simulink model "successPIDClosedLoop20picont"  (R2023b)
settings: Solver=FixedStepAuto  StartTime=0.0  StopTime=inf  RelTol=1e-3  EnableMultiTasking=on
libraries: arduinolib x5, simulink x1, arduinosensorlib x1, slpidlib x1
(part 2 of 3)

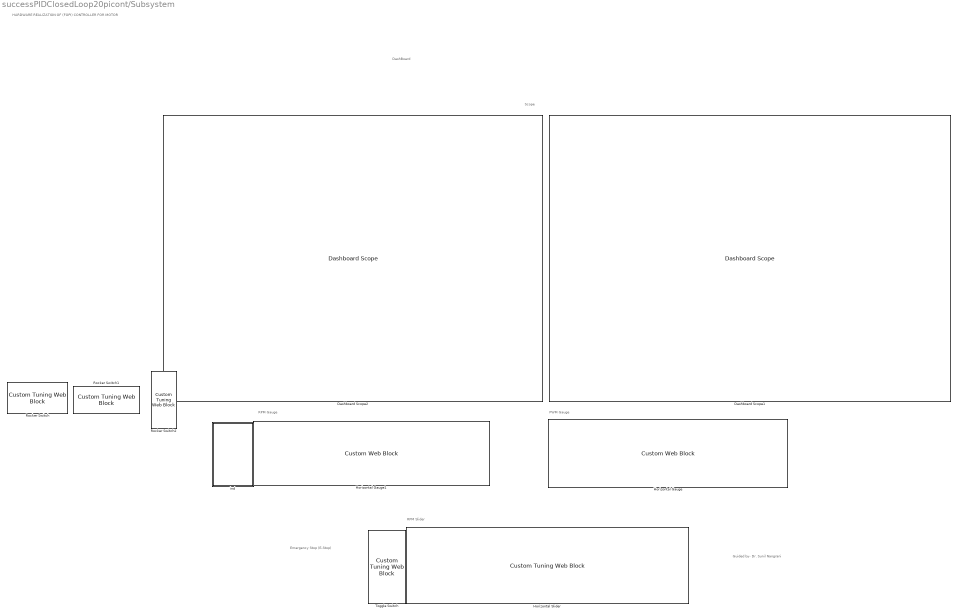
== system successPIDClosedLoop20picont/Subsystem ==
  note: PWM Gauge
  note: RPM Slider
  note: RPM Gauge
  note: Emergency Stop (E-Stop)
  note: DashBoard
  note: Scope
  note: Guided by-
      | Dr. Sunil Nangrani
  note: HARDWARE REALIZATION OF (FOPI) CONTROLLER FOR MOTOR
  Dashboard Scope1 : DashboardScope  UpdateMode=Scroll
  Dashboard Scope2 : DashboardScope  UpdateMode=Scroll
  Horizontal Gauge : CustomWebBlock  LabelPosition=Hide  ShowInitialText=on  Configuration="{\"components\":[{\"name\":\"LinearScaleComponent\",\"settings\":{\"bounds\":{\"max\":1000,\"min\":0,\"tickInterval\":\"auto\"},\"internalTickHeightScaleFactor\":0.5,\"labelColor\":[255,255,200],\"labelFont\":{\"font\":\"Arial\",\"fontSize\":12},\"labelOffset\":0.05,\"labelTransparency\":1,\"needleImage\":{\"size\":[21,75],\"src\":\"data:image\\/svg+xml;base64,PHN2ZyB4bWxucz0iaHR0cDovL3d3dy53My5vcmcvMjAwMC9zdmciIHhtbG5zOnhsaW5rPSJodHRwOi8vd3d3LnczLm9yZy8xOTk5L3hsaW5rIiB2aWV3Qm94PSIwIDAgMjEgNzUiPjxkZWZzPjxzdHlsZT4uY2xzLTF7ZmlsbDpub25lO30uY2xzLTJ7aXNvbGF0aW9uOmlzb2xhdGU7fS5jbHMtM3tjbGlwLXBhdGg6dXJsKCNjbGlwLXBhdGgpO30uY2xzLTR7b3BhY2l0eTowLjM7bWl4LWJsZW5kLW1vZGU6bXVsdGlwbHk7fS5jbHMtNXtmaWxsOiNlYjI2Mjk7fTwvc3R5bGU+PGNsaXBQYXRoIGlkPSJjbGlwLXBhdGgiIHRyYW5zZm9y ...(+1928 chars)\",\"srcOrientation\":\"Right\"},\"needleOffset\":[0.046142754145638065,0.04208955223880597],\"needleSize\":{\"height\":0.7998846597462514,\"width\":0.12797982885085574},\"position\":[0.06969246031746032,0.01995798319327731,0.9641544117647058,0.7998511904761905],\"referencePoint\":\"auto\",\"scaleColors\":[],\"scaleColorsSize\":0.2,\"scaleDirection\":\"LR\",\"showLabels\":1,\"showMinorTicks\":0,\"showSpanLine\":1,\"showTicks\":1,\"tickColor\":[252,252,197],\"tickTransparency\":1,\"valueBarColor\":[23,89,176],\"valueBarOffset\":0,\"valueBarSize\":0.23,\"valueBarTransparency\":1}},{\"name\":\"BackgroundImageComponent\",\"settings\":{\"image\":{\"size\":[380,101],\"src\":\"data:image\\/svg+xml;base64,PHN2ZyBpZD0iZnJhbWUiIHhtbG5zPSJodHRwOi8vd3d3LnczLm9yZy8yMDAwL3N2ZyIgeG1sbnM6eGxpbms9Imh0dHA6Ly93d3cudzMub3JnLzE5OTkveGxpbmsiIHZpZXdCb3g9IjAgMCAzODAgMTAxIj48ZGVmcz48c3R5bGU+LmNscy0xe2ZpbGw6IzAwMmI0Mjt9LmNscy0ye2ZpbGw6IzQyNzA4Mjt9LmNscy0ze2ZpbGw6dXJsKCNyYWRpYWwtZ3JhZGllbnQpO308L3N0eWxlPjxyYWRpYWxHcmFkaWVudCBpZD0icmFkaWFsLWdyYWRpZW50IiBjeD0iMTkwIiBjeT0iNTAuNSIgcj0iMjY5LjIxIiBncmFkaWVudFVuaXRzPSJ1c2VyU3BhY2VPblVzZSI+PHN0b3Agb2Zmc2V0PSIwLjAxIiBzdG9wLWNvbG9yPSIjM2U0ZjU4Ii8+PHN0b3Agb2Zmc2V0PSIwLjA2IiBzdG9wLWNvbG9yPSIjNDQ1NzYxIi8+PHN0b3Agb2Zmc2V0PSIwLjE1IiBzdG9wLWNvbG9yPSIjNTU2YTc2Ii8+PHN0b3Agb2Zmc2V0PSIwLjI1IiBzdG9wLWNvbG9yPSIjNmQ4ODk1Ii8+PHN0b3Agb2Zmc2V0PSIwLjM4IiBzdG9wLWNvbG9yPSIjOGZiMmMzIi8+PHN0b3Agb2Zmc2V0PSIwLjUyIiBzdG9wLWNvbG9yPSIjYjZlNGZhIi8+PHN0b3Agb2Zmc2V0PSIxIiBzdG9wLWNvbG9yPSIjMTU0NjU3Ii8+PC9yYWRpYWxHcmFkaWVudD48L2RlZnM+PGcgaWQ9IkxheWVyXzIiIGRhdGEtbmFtZT0iTGF5ZXIgMiI+PGcgaWQ9IkxheWVyXzEtMiIgZGF0YS1uYW1lPSJMYXllciAxLTIiPjxyZWN0IGlkPSJyZWN0MTAzNiIgY2xhc3M9ImNscy0xIiB4PSIxMSIgeT0iMTEiIHdpZHRoPSIzNTgiIGhlaWdodD0iNzkiLz48cGF0aCBpZD0icGF0aDEwMzgiIGNsYXNzPSJjbHMtMiIgZD0iTTgsOFY5M0gzNzJWOFpNMzY5LDkwSDExVjExSDM2OVoiLz48cGF0aCBpZD0icGF0aDEwNDAiIGNsYXNzPSJjbHMtMyIgZD0iTTAsMFYxMDFIMzgwVjBaTTM3Miw5M0g4VjhIMzcyWiIvPjwvZz48L2c+PC9zdmc+\",\"srcOrientation\":\"horizontal\"},\"position\":[0,0,1,1],\"scaleMode\":\"0\"}},{\"name\":\"ForegroundImageComponent\",\"settings\":{\"image\":{\"size\":[0,0],\"src\":\"default\",\"srcOrientation\":[]},\"isForeground\":1,\"position\":[0,0,1,1],\"scaleMode\":\"0\"}}],\"settings\":{\"BindingType\":\"signal\",\"backgroundColor\":[0,0,0,\"1\"],\"backgroundOffset\":0,\"backgroundOpacity\":1,\"fixedAspectRatio\":\"on\",\"orientation\":\"horizontal\",\"showBackgroundColor\":false,\"value\":0,\"version\":\"R2023a\"},\"type\":\"LinearGauge\"}"
  Horizontal Gauge1 : CustomWebBlock  LabelPosition=Hide  ShowInitialText=on  Configuration="{\"components\":[{\"name\":\"LinearScaleComponent\",\"settings\":{\"bounds\":{\"max\":1000,\"min\":0,\"tickInterval\":\"auto\"},\"internalTickHeightScaleFactor\":0.5,\"labelColor\":[255,255,200],\"labelFont\":{\"font\":\"Arial\",\"fontSize\":12},\"labelOffset\":0.05,\"labelTransparency\":1,\"needleImage\":{\"size\":[21,75],\"src\":\"data:image\\/svg+xml;base64,PHN2ZyB4bWxucz0iaHR0cDovL3d3dy53My5vcmcvMjAwMC9zdmciIHhtbG5zOnhsaW5rPSJodHRwOi8vd3d3LnczLm9yZy8xOTk5L3hsaW5rIiB2aWV3Qm94PSIwIDAgMjEgNzUiPjxkZWZzPjxzdHlsZT4uY2xzLTF7ZmlsbDpub25lO30uY2xzLTJ7aXNvbGF0aW9uOmlzb2xhdGU7fS5jbHMtM3tjbGlwLXBhdGg6dXJsKCNjbGlwLXBhdGgpO30uY2xzLTR7b3BhY2l0eTowLjM7bWl4LWJsZW5kLW1vZGU6bXVsdGlwbHk7fS5jbHMtNXtmaWxsOiNlYjI2Mjk7fTwvc3R5bGU+PGNsaXBQYXRoIGlkPSJjbGlwLXBhdGgiIHRyYW5zZm9y ...(+1928 chars)\",\"srcOrientation\":\"Right\"},\"needleOffset\":[0.046142754145638065,0.04208955223880597],\"needleSize\":{\"height\":0.7998846597462514,\"width\":0.12797982885085574},\"position\":[0.06969246031746032,0.01995798319327731,0.9641544117647058,0.7998511904761905],\"referencePoint\":\"auto\",\"scaleColors\":[],\"scaleColorsSize\":0.2,\"scaleDirection\":\"LR\",\"showLabels\":1,\"showMinorTicks\":0,\"showSpanLine\":1,\"showTicks\":1,\"tickColor\":[252,252,197],\"tickTransparency\":1,\"valueBarColor\":[23,89,176],\"valueBarOffset\":0,\"valueBarSize\":0.23,\"valueBarTransparency\":1}},{\"name\":\"BackgroundImageComponent\",\"settings\":{\"image\":{\"size\":[380,101],\"src\":\"data:image\\/svg+xml;base64,PHN2ZyBpZD0iZnJhbWUiIHhtbG5zPSJodHRwOi8vd3d3LnczLm9yZy8yMDAwL3N2ZyIgeG1sbnM6eGxpbms9Imh0dHA6Ly93d3cudzMub3JnLzE5OTkveGxpbmsiIHZpZXdCb3g9IjAgMCAzODAgMTAxIj48ZGVmcz48c3R5bGU+LmNscy0xe2ZpbGw6IzAwMmI0Mjt9LmNscy0ye2ZpbGw6IzQyNzA4Mjt9LmNscy0ze2ZpbGw6dXJsKCNyYWRpYWwtZ3JhZGllbnQpO308L3N0eWxlPjxyYWRpYWxHcmFkaWVudCBpZD0icmFkaWFsLWdyYWRpZW50IiBjeD0iMTkwIiBjeT0iNTAuNSIgcj0iMjY5LjIxIiBncmFkaWVudFVuaXRzPSJ1c2VyU3BhY2VPblVzZSI+PHN0b3Agb2Zmc2V0PSIwLjAxIiBzdG9wLWNvbG9yPSIjM2U0ZjU4Ii8+PHN0b3Agb2Zmc2V0PSIwLjA2IiBzdG9wLWNvbG9yPSIjNDQ1NzYxIi8+PHN0b3Agb2Zmc2V0PSIwLjE1IiBzdG9wLWNvbG9yPSIjNTU2YTc2Ii8+PHN0b3Agb2Zmc2V0PSIwLjI1IiBzdG9wLWNvbG9yPSIjNmQ4ODk1Ii8+PHN0b3Agb2Zmc2V0PSIwLjM4IiBzdG9wLWNvbG9yPSIjOGZiMmMzIi8+PHN0b3Agb2Zmc2V0PSIwLjUyIiBzdG9wLWNvbG9yPSIjYjZlNGZhIi8+PHN0b3Agb2Zmc2V0PSIxIiBzdG9wLWNvbG9yPSIjMTU0NjU3Ii8+PC9yYWRpYWxHcmFkaWVudD48L2RlZnM+PGcgaWQ9IkxheWVyXzIiIGRhdGEtbmFtZT0iTGF5ZXIgMiI+PGcgaWQ9IkxheWVyXzEtMiIgZGF0YS1uYW1lPSJMYXllciAxLTIiPjxyZWN0IGlkPSJyZWN0MTAzNiIgY2xhc3M9ImNscy0xIiB4PSIxMSIgeT0iMTEiIHdpZHRoPSIzNTgiIGhlaWdodD0iNzkiLz48cGF0aCBpZD0icGF0aDEwMzgiIGNsYXNzPSJjbHMtMiIgZD0iTTgsOFY5M0gzNzJWOFpNMzY5LDkwSDExVjExSDM2OVoiLz48cGF0aCBpZD0icGF0aDEwNDAiIGNsYXNzPSJjbHMtMyIgZD0iTTAsMFYxMDFIMzgwVjBaTTM3Miw5M0g4VjhIMzcyWiIvPjwvZz48L2c+PC9zdmc+\",\"srcOrientation\":\"horizontal\"},\"position\":[0,0,1,1],\"scaleMode\":\"0\"}},{\"name\":\"ForegroundImageComponent\",\"settings\":{\"image\":{\"size\":[0,0],\"src\":\"default\",\"srcOrientation\":[]},\"isForeground\":1,\"position\":[0,0,1,1],\"scaleMode\":\"0\"}}],\"settings\":{\"BindingType\":\"signal\",\"backgroundColor\":[0,0,0,\"1\"],\"backgroundOffset\":0,\"backgroundOpacity\":1,\"fixedAspectRatio\":\"on\",\"orientation\":\"horizontal\",\"showBackgroundColor\":false,\"value\":0,\"version\":\"R2023a\"},\"type\":\"LinearGauge\"}"
  Horizontal Slider : CustomTuningWebBlock  LabelPosition=Hide  ShowInitialText=on  Configuration="{\"components\":[{\"name\":\"LinearScaleComponent\",\"settings\":{\"bounds\":{\"max\":1000,\"min\":0,\"tickInterval\":\"auto\"},\"internalTickHeightScaleFactor\":0.5,\"labelColor\":[255,255,200],\"labelFont\":{\"font\":\"Arial\",\"fontSize\":12},\"labelOffset\":0.05,\"labelTransparency\":1,\"needleImage\":{\"size\":[596,842],\"src\":\"data:image\\/svg+xml;base64,PD94bWwgdmVyc2lvbj0iMS4wIiBlbmNvZGluZz0idXRmLTgiPz4NCjwhLS0gR2VuZXJhdG9yOiBBZG9iZSBJbGx1c3RyYXRvciAyNS4wLjAsIFNWRyBFeHBvcnQgUGx1Zy1JbiAuIFNWRyBWZXJzaW9uOiA2LjAwIEJ1aWxkIDApICAtLT4NCjxzdmcgdmVyc2lvbj0iMS4xIg0KCSBpZD0ic3ZnOCIgeG1sbnM6Y2M9Imh0dHA6Ly9jcmVhdGl2ZWNvbW1vbnMub3JnL25zIyIgeG1sbnM6ZGM9Imh0dHA6Ly9wdXJsLm9yZy9kYy9lbGVtZW50cy8xLjEvIiB4bWxuczppbmtzY2FwZT0iaHR0cDovL3d3dy5pbmtzY2FwZS5vcmcvbmFtZXNw ...(+2420 chars)\",\"srcOrientation\":\"Right\"},\"needleOffset\":[-0.8044596912521441,-0.0642123287671233],\"needleSize\":{\"height\":0.4337797619047619,\"width\":0.07668067226890757},\"position\":[0.2829861111111111,0.04398634453781513,0.9196428571428571,0.6088789682539683],\"referencePoint\":\"auto\",\"scaleColors\":[],\"scaleColorsSize\":0.2,\"scaleDirection\":\"LR\",\"showLabels\":1,\"showMinorTicks\":0,\"showSpanLine\":1,\"showTicks\":1,\"tickColor\":[252,252,197],\"tickTransparency\":1,\"valueBarColor\":[0,114,189],\"valueBarOffset\":-0.27,\"valueBarSize\":0.1,\"valueBarTransparency\":1}},{\"name\":\"BackgroundImageComponent\",\"settings\":{\"image\":{\"size\":[380,101],\"src\":\"data:image\\/svg+xml;base64,PHN2ZyB4bWxucz0iaHR0cDovL3d3dy53My5vcmcvMjAwMC9zdmciIHhtbG5zOnhsaW5rPSJodHRwOi8vd3d3LnczLm9yZy8xOTk5L3hsaW5rIiB2aWV3Qm94PSIwIDAgMzgwIDEwMSI+PGRlZnM+PHN0eWxlPi5jbHMtMXtmaWxsOiMwMDJiNDI7fS5jbHMtMntmaWxsOiM0MjcwODI7fS5jbHMtM3tmaWxsOnVybCgjcmFkaWFsLWdyYWRpZW50KTt9LmNscy00e2ZpbGw6I2M4YzhjODtzdHJva2U6IzAwMDt9PC9zdHlsZT48cmFkaWFsR3JhZGllbnQgaWQ9InJhZGlhbC1ncmFkaWVudCIgY3g9IjE5MCIgY3k9IjUwLjUiIHI9IjI2OS4yMSIgZ3JhZGllbnRVbml0cz0idXNlclNwYWNlT25Vc2UiPjxzdG9wIG9mZnNldD0iMC4wMSIgc3RvcC1jb2xvcj0iIzNlNGY1OCIvPjxzdG9wIG9mZnNldD0iMC4wNiIgc3RvcC1jb2xvcj0iIzQ0NTc2MSIvPjxzdG9wIG9mZnNldD0iMC4xNSIgc3RvcC1jb2xvcj0iIzU1NmE3NiIvPjxzdG9wIG9mZnNldD0iMC4yNSIgc3RvcC1jb2xvcj0iIzZkODg5NSIvPjxzdG9wIG9mZnNldD0iMC4zOCIgc3RvcC1jb2xvcj0iIzhmYjJjMyIvPjxzdG9wIG9mZnNldD0iMC41MiIgc3RvcC1jb2xvcj0iI2I2ZTRmYSIvPjxzdG9wIG9mZnNldD0iMSIgc3RvcC1jb2xvcj0iIzE1NDY1NyIvPjwvcmFkaWFsR3JhZGllbnQ+PC9kZWZzPjxnIGlkPSJmcmFtZSI+PGcgaWQ9IkxheWVyXzIiIGRhdGEtbmFtZT0iTGF5ZXIgMiI+PGcgaWQ9IkxheWVyXzEtMiIgZGF0YS1uYW1lPSJMYXllciAxLTIiPjxyZWN0IGlkPSJyZWN0MTAzNiIgY2xhc3M9ImNscy0xIiB4PSIxMSIgeT0iMTEiIHdpZHRoPSIzNTgiIGhlaWdodD0iNzkiLz48cGF0aCBpZD0icGF0aDEwMzgiIGNsYXNzPSJjbHMtMiIgZD0iTTgsOFY5M0gzNzJWOFpNMzY5LDkwSDExVjExSDM2OVoiLz48cGF0aCBpZD0icGF0aDEwNDAiIGNsYXNzPSJjbHMtMyIgZD0iTTAsMFYxMDFIMzgwVjBaTTM3Miw5M0g4VjhIMzcyWiIvPjwvZz48L2c+PC9nPjxnIGlkPSJ0cmFjayI+PHBhdGggaWQ9InJlY3QxNjExIiBjbGFzcz0iY2xzLTQiIGQ9Ik0zMy4zNywyNi41OUgzNDYuNjNjNCwwLDcuMjUsMi42LDcuMjUsNS44MWgwYzAsMy4yMS0zLjI1LDUuODItNy4yNSw1LjgySDMzLjM3Yy00LDAtNy4yNS0yLjYxLTcuMjUtNS44MmgwQzI2LjEyLDI5LjE5LDI5LjM3LDI2LjU5LDMzLjM3LDI2LjU5WiIvPjwvZz48L3N2Zz4=\",\"srcOrientation\":\"horizontal\"},\"position\":[0,0,1,1],\"scaleMode\":\"0\"}},{\"name\":\"ForegroundImageComponent\",\"settings\":{\"image\":{\"size\":[0,0],\"src\":\"default\",\"srcOrientation\":[]},\"isForeground\":1,\"position\":[0,0,1,1],\"scaleMode\":\"0\"}}],\"settings\":{\"BindingType\":\"param\",\"aspectRatio\":3.7777777777777777,\"backgroundColor\":[0,0,0,\"1\"],\"backgroundOffset\":0,\"backgroundOpacity\":1,\"fixedAspectRatio\":\"on\",\"foregroundColor\":[252,252,196],\"orientation\":\"horizontal\",\"showBackgroundColor\":false,\"value\":0,\"version\":\"R2023a\"},\"type\":\"LinearGauge\"}"
  Rocker Switch : CustomTuningWebBlock  LabelPosition=Hide  ShowInitialText=on  Configuration="{\"components\":[{\"name\":\"CustomSwitchStateComponent\",\"settings\":{\"position\":[0,0,1,1],\"states\":[{\"HitRegion\":{\"position\":[0,0,0.5,1]},\"Image\":{\"position\":[0.13,0,1,0.75],\"size\":[1,0.75],\"src\":\"data:image\\/svg+xml;base64,PHN2ZyB4bWxucz0iaHR0cDovL3d3dy53My5vcmcvMjAwMC9zdmciIHhtbG5zOnhsaW5rPSJodHRwOi8vd3d3LnczLm9yZy8xOTk5L3hsaW5rIiB2aWV3Qm94PSIwIDAgNzUgMjQuOCI+PGRlZnM+PHN0eWxlPi5jbHMtMXtmaWxsOnVybCgjcmFkaWFsLWdyYWRpZW50KTt9LmNscy0ye2ZpbGw6dXJsKCNyYWRpYWwtZ3JhZGllbnQtMik7fS5jbHMtM3tzdHJva2U6I2IyMDAwMDtzdHJva2Utd2lkdGg6MC4yNXB4O2ZpbGw6dXJsKCNsaW5lYXItZ3JhZGllbnQpO30uY2xzLTR7ZmlsbDp1cmwoI2xpbmVhci1ncmFkaWVudC0yKTt9LmNs ...(+3576 chars)\",\"srcOrientation\":\"Right\"},\"Label\":{\"color\":[0.5019607843137255,0.5019607843137255,0.5019607843137255],\"icon\":{\"size\":[0,0],\"src\":[],\"srcOrientation\":\"Right\"},\"iconPlacement\":\"left\",\"opacity\":1,\"position\":[0.5,0.07999999999999996],\"show\":true,\"text\":{\"content\":\"Off\",\"font\":\"Helvetica\",\"fontSize\":14}},\"Value\":0},{\"HitRegion\":{\"position\":[0,0.5,0.5,1]},\"Image\":{\"position\":[0.13,0,1,0.75],\"size\":[1,0.75],\"src\":\"data:image\\/svg+xml;base64,PHN2ZyB4bWxucz0iaHR0cDovL3d3dy53My5vcmcvMjAwMC9zdmciIHhtbG5zOnhsaW5rPSJodHRwOi8vd3d3LnczLm9yZy8xOTk5L3hsaW5rIiB2aWV3Qm94PSIwIDAgNzUgMjQuOCI+PGRlZnM+PHN0eWxlPi5jbHMtMXtmaWxsOnVybCgjcmFkaWFsLWdyYWRpZW50KTt9LmNscy0ye2ZpbGw6dXJsKCNyYWRpYWwtZ3JhZGllbnQtMik7fS5jbHMtM3tzdHJva2U6I2IyMDAwMDtzdHJva2Utd2lkdGg6MC4yNXB4O2ZpbGw6dXJsKCNsaW5lYXItZ3JhZGllbnQpO30uY2xzLTR7ZmlsbDp1cmwoI2xpbmVhci1ncmFkaWVudC0yKTt9LmNs ...(+3520 chars)\",\"srcOrientation\":\"Right\"},\"Label\":{\"color\":[0.5019607843137255,0.5019607843137255,0.5019607843137255],\"icon\":{\"size\":[0,0],\"src\":[],\"srcOrientation\":\"Right\"},\"iconPlacement\":\"left\",\"opacity\":1,\"position\":[0.5,0.92],\"show\":true,\"text\":{\"content\":\"On\",\"font\":\"Helvetica\",\"fontSize\":14}},\"Value\":1}]}},{\"name\":\"BackgroundImageComponent\",\"settings\":{\"image\":{\"size\":[155,70],\"src\":\"default\",\"srcOrientation\":\"Right\"},\"position\":[0,0,1,1],\"scaleMode\":\"0\"}},{\"name\":\"ForegroundImageComponent\",\"settings\":{\"image\":{\"size\":[0,0],\"src\":\"default\",\"srcOrientation\":[]},\"isForeground\":1,\"position\":[0,0,1,1],\"scaleMode\":\"0\"}}],\"settings\":{\"BindingType\":\"param\",\"backgroundColor\":[0,0,255,\"1\"],\"backgroundOffset\":0.14,\"fixedAspectRatio\":\"on\",\"foregroundColor\":[234,234,234],\"showBackgroundColor\":false,\"variant\":\"rocker\",\"version\":\"R2023a\"},\"type\":\"Switch\"}"
  Rocker Switch1 : CustomTuningWebBlock  LabelPosition=Hide  ShowInitialText=on  Configuration="{\"components\":[{\"name\":\"CustomSwitchStateComponent\",\"settings\":{\"position\":[0,0,1,1],\"states\":[{\"HitRegion\":{\"position\":[0,0.5,0.5,1]},\"Image\":{\"position\":[0.12,0,1,0.75],\"size\":[1,0.75],\"src\":\"data:image\\/svg+xml;base64,PHN2ZyB4bWxucz0iaHR0cDovL3d3dy53My5vcmcvMjAwMC9zdmciIHhtbG5zOnhsaW5rPSJodHRwOi8vd3d3LnczLm9yZy8xOTk5L3hsaW5rIiB2aWV3Qm94PSIwIDAgNzUgMjQuOCI+PGRlZnM+PHN0eWxlPi5jbHMtMXtmaWxsOnVybCgjcmFkaWFsLWdyYWRpZW50KTt9LmNscy0ye2ZpbGw6dXJsKCNyYWRpYWwtZ3JhZGllbnQtMik7fS5jbHMtM3tzdHJva2U6I2IyMDAwMDtzdHJva2Utd2lkdGg6MC4yNXB4O2ZpbGw6dXJsKCNsaW5lYXItZ3JhZGllbnQpO30uY2xzLTR7ZmlsbDp1cmwoI2xpbmVhci1ncmFkaWVudC0yKTt9LmNs ...(+3576 chars)\",\"srcOrientation\":\"Right\"},\"Label\":{\"color\":[0.5019607843137255,0.5019607843137255,0.5019607843137255],\"icon\":{\"size\":[0,0],\"src\":[],\"srcOrientation\":\"Right\"},\"iconPlacement\":\"left\",\"opacity\":1,\"position\":[0.5,0.92],\"show\":true,\"text\":{\"content\":\"Off\",\"font\":\"Helvetica\",\"fontSize\":14}},\"Value\":0},{\"HitRegion\":{\"position\":[0,0,0.5,1]},\"Image\":{\"position\":[0.12,0,1,0.75],\"size\":[1,0.75],\"src\":\"data:image\\/svg+xml;base64,PHN2ZyB4bWxucz0iaHR0cDovL3d3dy53My5vcmcvMjAwMC9zdmciIHhtbG5zOnhsaW5rPSJodHRwOi8vd3d3LnczLm9yZy8xOTk5L3hsaW5rIiB2aWV3Qm94PSIwIDAgNzUgMjQuOCI+PGRlZnM+PHN0eWxlPi5jbHMtMXtmaWxsOnVybCgjcmFkaWFsLWdyYWRpZW50KTt9LmNscy0ye2ZpbGw6dXJsKCNyYWRpYWwtZ3JhZGllbnQtMik7fS5jbHMtM3tzdHJva2U6I2IyMDAwMDtzdHJva2Utd2lkdGg6MC4yNXB4O2ZpbGw6dXJsKCNsaW5lYXItZ3JhZGllbnQpO30uY2xzLTR7ZmlsbDp1cmwoI2xpbmVhci1ncmFkaWVudC0yKTt9LmNs ...(+3520 chars)\",\"srcOrientation\":\"Right\"},\"Label\":{\"color\":[0.5019607843137255,0.5019607843137255,0.5019607843137255],\"icon\":{\"size\":[0,0],\"src\":[],\"srcOrientation\":\"Right\"},\"iconPlacement\":\"left\",\"opacity\":1,\"position\":[0.5,0.07999999999999996],\"show\":true,\"text\":{\"content\":\"On\",\"font\":\"Helvetica\",\"fontSize\":14}},\"Value\":1}]}},{\"name\":\"BackgroundImageComponent\",\"settings\":{\"image\":{\"size\":[155,70],\"src\":\"default\",\"srcOrientation\":\"Right\"},\"position\":[0,0,1,1],\"scaleMode\":\"0\"}},{\"name\":\"ForegroundImageComponent\",\"settings\":{\"image\":{\"size\":[0,0],\"src\":\"default\",\"srcOrientation\":[]},\"isForeground\":1,\"position\":[0,0,1,1],\"scaleMode\":\"0\"}}],\"settings\":{\"BindingType\":\"param\",\"backgroundColor\":[0,0,255,\"1\"],\"backgroundOffset\":0.14,\"fixedAspectRatio\":\"on\",\"foregroundColor\":[234,234,234],\"showBackgroundColor\":false,\"variant\":\"rocker\",\"version\":\"R2023a\"},\"type\":\"Switch\"}"
  Rocker Switch2 : CustomTuningWebBlock  LabelPosition=Hide  ShowInitialText=on  Configuration="{\"components\":[{\"name\":\"CustomSwitchStateComponent\",\"settings\":{\"position\":[0,0,1,1],\"states\":[{\"HitRegion\":{\"position\":[0,0,1,0.5]},\"Image\":{\"position\":[0,0.12,0.75,1],\"size\":[0.75,1],\"src\":\"data:image\\/svg+xml;base64,PHN2ZyB4bWxucz0iaHR0cDovL3d3dy53My5vcmcvMjAwMC9zdmciIHhtbG5zOnhsaW5rPSJodHRwOi8vd3d3LnczLm9yZy8xOTk5L3hsaW5rIiB2aWV3Qm94PSIwIDAgNzUgMjQuOCI+PGRlZnM+PHN0eWxlPi5jbHMtMXtmaWxsOnVybCgjcmFkaWFsLWdyYWRpZW50KTt9LmNscy0ye2ZpbGw6dXJsKCNyYWRpYWwtZ3JhZGllbnQtMik7fS5jbHMtM3tzdHJva2U6I2IyMDAwMDtzdHJva2Utd2lkdGg6MC4yNXB4O2ZpbGw6dXJsKCNsaW5lYXItZ3JhZGllbnQpO30uY2xzLTR7ZmlsbDp1cmwoI2xpbmVhci1ncmFkaWVudC0yKTt9LmNs ...(+3576 chars)\",\"srcOrientation\":\"Right\"},\"Label\":{\"color\":[0.5019607843137255,0.5019607843137255,0.5019607843137255],\"icon\":{\"size\":[0,0],\"src\":[],\"srcOrientation\":\"Right\"},\"iconPlacement\":\"left\",\"opacity\":1,\"position\":[0.08,0.5],\"show\":true,\"text\":{\"content\":\"Off\",\"font\":\"Helvetica\",\"fontSize\":14}},\"Value\":0},{\"HitRegion\":{\"position\":[0.5,0,1,0.5]},\"Image\":{\"position\":[0,0.12,0.75,1],\"size\":[0.75,1],\"src\":\"data:image\\/svg+xml;base64,PHN2ZyB4bWxucz0iaHR0cDovL3d3dy53My5vcmcvMjAwMC9zdmciIHhtbG5zOnhsaW5rPSJodHRwOi8vd3d3LnczLm9yZy8xOTk5L3hsaW5rIiB2aWV3Qm94PSIwIDAgNzUgMjQuOCI+PGRlZnM+PHN0eWxlPi5jbHMtMXtmaWxsOnVybCgjcmFkaWFsLWdyYWRpZW50KTt9LmNscy0ye2ZpbGw6dXJsKCNyYWRpYWwtZ3JhZGllbnQtMik7fS5jbHMtM3tzdHJva2U6I2IyMDAwMDtzdHJva2Utd2lkdGg6MC4yNXB4O2ZpbGw6dXJsKCNsaW5lYXItZ3JhZGllbnQpO30uY2xzLTR7ZmlsbDp1cmwoI2xpbmVhci1ncmFkaWVudC0yKTt9LmNs ...(+3520 chars)\",\"srcOrientation\":\"Right\"},\"Label\":{\"color\":[0.5019607843137255,0.5019607843137255,0.5019607843137255],\"icon\":{\"size\":[0,0],\"src\":[],\"srcOrientation\":\"Right\"},\"iconPlacement\":\"left\",\"opacity\":1,\"position\":[0.92,0.5],\"show\":true,\"text\":{\"content\":\"On\",\"font\":\"Helvetica\",\"fontSize\":14}},\"Value\":1}]}},{\"name\":\"BackgroundImageComponent\",\"settings\":{\"image\":{\"size\":[155,70],\"src\":\"default\",\"srcOrientation\":\"Right\"},\"position\":[0,0,1,1],\"scaleMode\":\"0\"}},{\"name\":\"ForegroundImageComponent\",\"settings\":{\"image\":{\"size\":[0,0],\"src\":\"default\",\"srcOrientation\":[]},\"isForeground\":1,\"position\":[0,0,1,1],\"scaleMode\":\"0\"}}],\"settings\":{\"BindingType\":\"param\",\"backgroundColor\":[0,0,255,\"1\"],\"backgroundOffset\":0.14,\"fixedAspectRatio\":\"on\",\"foregroundColor\":[234,234,234],\"showBackgroundColor\":false,\"variant\":\"rocker\",\"version\":\"R2023a\"},\"type\":\"Switch\"}"
  Toggle Switch : CustomTuningWebBlock  LabelPosition=Hide  ShowInitialText=on  Configuration="{\"components\":[{\"name\":\"CustomSwitchStateComponent\",\"settings\":{\"position\":[0,0,1,1],\"showAllLabels\":1,\"states\":[{\"HitRegion\":{\"position\":[0.5,0,1,0.5]},\"Image\":{\"position\":[0,0.24928571428571428,0.5014285714285714,1],\"size\":[0.5014285714285714,1],\"src\":\"data:image\\/svg+xml;base64,PHN2ZyB4bWxucz0iaHR0cDovL3d3dy53My5vcmcvMjAwMC9zdmciIHhtbG5zOnhsaW5rPSJodHRwOi8vd3d3LnczLm9yZy8xOTk5L3hsaW5rIiB2aWV3Qm94PSIwIDAgMzguMDQgMTUwIj48ZGVmcz48c3R5bGU+LmNscy0xe2ZpbGw6dXJsKCNyYWRpYWwtZ3JhZGllbnQpO30uY2xzLTJ7ZmlsbDp1cmwoI3JhZGlhbC1ncmFkaWVudC0yKTt9LmNscy0ze2ZpbGw6dXJsKCNXaGl0ZV9CbGFjayk7fS5jbHMtNHtmaWxsOnVybCgjcmFkaWFsLWdyYWRpZW50LTMpO30uY2xzLTV7ZmlsbDojNWI1YjViO30uY2xzLTZ7ZmlsbDp1cmwoI3Jh ...(+3556 chars)\",\"srcOrientation\":\"Right\"},\"Label\":{\"color\":[0.8980392156862745,0,0],\"icon\":{\"size\":[0,0],\"src\":[],\"srcOrientation\":\"Right\"},\"iconPlacement\":\"left\",\"opacity\":1,\"position\":[0.92,0.5],\"show\":true,\"text\":{\"content\":\"Off\",\"font\":\"Helvetica\",\"fontSize\":14}},\"Value\":0},{\"HitRegion\":{\"position\":[0,0,1,0.5]},\"Image\":{\"position\":[0,0.24928571428571428,0.5014285714285714,1],\"size\":[0.5014285714285714,1],\"src\":\"data:image\\/svg+xml;base64,PHN2ZyB4bWxucz0iaHR0cDovL3d3dy53My5vcmcvMjAwMC9zdmciIHhtbG5zOnhsaW5rPSJodHRwOi8vd3d3LnczLm9yZy8xOTk5L3hsaW5rIiB2aWV3Qm94PSIwIDAgMzguMDQgMTUwIj48ZGVmcz48c3R5bGU+LmNscy0xe2ZpbGw6dXJsKCNyYWRpYWwtZ3JhZGllbnQpO30uY2xzLTJ7ZmlsbDp1cmwoI3JhZGlhbC1ncmFkaWVudC0yKTt9LmNscy0ze2ZpbGw6dXJsKCNXaGl0ZV9CbGFjayk7fS5jbHMtNHtmaWxsOnVybCgjcmFkaWFsLWdyYWRpZW50LTMpO30uY2xzLTV7ZmlsbDojNWI1YjViO30uY2xzLTZ7ZmlsbDp1cmwoI3Jh ...(+3628 chars)\",\"srcOrientation\":\"Right\"},\"Label\":{\"color\":[0.8980392156862745,0,0],\"icon\":{\"size\":[0,0],\"src\":[],\"srcOrientation\":\"Right\"},\"iconPlacement\":\"left\",\"opacity\":1,\"position\":[0.08,0.5],\"show\":true,\"text\":{\"content\":\"On\",\"font\":\"Helvetica\",\"fontSize\":14}},\"Value\":1}]}},{\"name\":\"BackgroundImageComponent\",\"settings\":{\"image\":{\"size\":[70,135],\"src\":\"default\",\"srcOrientation\":\"Right\"},\"position\":[0,0,1,1],\"scaleMode\":\"0\"}},{\"name\":\"ForegroundImageComponent\",\"settings\":{\"image\":{\"size\":[0,0],\"src\":\"default\",\"srcOrientation\":[]},\"isForeground\":1,\"position\":[0,0,1,1],\"scaleMode\":\"0\"}}],\"settings\":{\"BindingType\":\"param\",\"backgroundColor\":[0,0,0],\"backgroundOffset\":0.14,\"fixedAspectRatio\":\"on\",\"foregroundColor\":[0,0,0],\"showBackgroundColor\":false,\"variant\":\"toggle\",\"version\":\"R2023a\"},\"type\":\"Switch\"}"
  ind : Subsystem
